simulink model "Inv_Pend_HInf3"  (R2023b)
settings: Solver=VariableStepAuto  StartTime=0.0  StopTime=35  RelTol=1e-3
undefined symbols (not defined in the file): A_, B_, C_, D
libraries: cstblocks x4
settings Model: Creator=DELL  LastModifiedBy=DELL

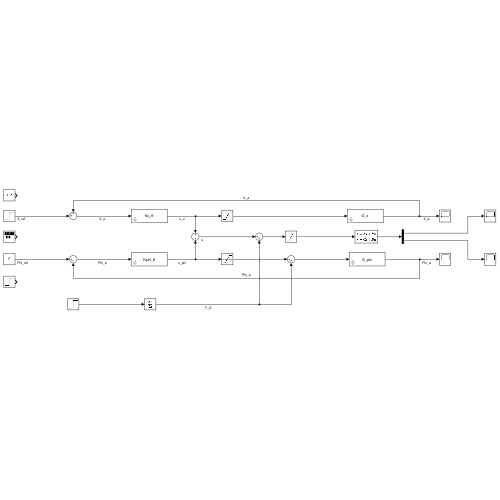
[thumbnail: Simulink's stored preview of the top-level diagram]
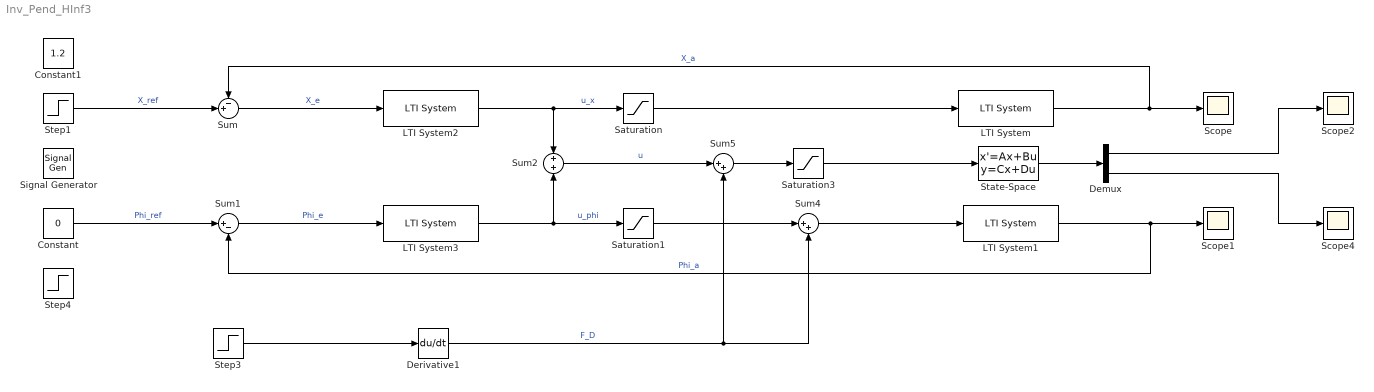
== system Inv_Pend_HInf3 ==
  Constant : Constant  Value=0
  Constant1 : Constant  Value=1.2
  Demux : Demux  Outputs=2
  Derivative1 : Derivative
  LTI System : cstblocks/LTI System  sys=G_x  IC=[]  PadeOrder=0
  LTI System1 : cstblocks/LTI System  sys=G_phi  IC=[]  PadeOrder=0
  LTI System2 : cstblocks/LTI System  sys=Kx_tf  IC=[]  PadeOrder=0
  LTI System3 : cstblocks/LTI System  sys=Kphi_tf  IC=[]  PadeOrder=0
  Saturation : Saturate  UpperLimit=50  LowerLimit=-50
  Saturation1 : Saturate  UpperLimit=50  LowerLimit=-50
  Saturation3 : Saturate  UpperLimit=50  LowerLimit=-50
  Scope{,1..2,4} (4 alike) : Scope
  Signal Generator : SignalGenerator  Amplitude=3
  State-Space : StateSpace  A=A_  B=B_  C=C_  D=D  InitialCondition=0
  Step1 : Step  SampleTime=0
  Step3 : Step  After=50  SampleTime=0
  Step4 : Step  After=1.4  SampleTime=0
  Sum : Sum  Inputs=-+|
  Sum1 : Sum  Inputs=|+-
  Sum2 : Sum  Inputs=+|+
  Sum4 : Sum  Inputs=|++
  Sum5 : Sum  Inputs=|++
  wires:
  LTI System/1 -> Sum/1, Scope/1  "X_a"
  LTI System1/1 -> Sum1/2, Scope1/1  "Phi_a"
  LTI System3/1 -> Saturation1/1, Sum2/2  "u_phi"
  LTI System2/1 -> Saturation/1, Sum2/1  "u_x"
  Sum/1 -> LTI System2/1  "X_e"
  Sum1/1 -> LTI System3/1  "Phi_e"
  Step3/1 -> Derivative1/1
  Derivative1/1 -> Sum5/2, Sum4/2  "F_D"
  Sum2/1 -> Sum5/1  "u"
  Sum4/1 -> LTI System1/1
  Saturation1/1 -> Sum4/1
  Step1/1 -> Sum/2  "X_ref"
  Constant/1 -> Sum1/1  "Phi_ref"
  Sum5/1 -> Saturation3/1
  State-Space/1 -> Demux/1
  Demux/1 -> Scope2/1
  Demux/2 -> Scope4/1
  Saturation3/1 -> State-Space/1
  Saturation/1 -> LTI System/1
